simulink model "Complete_Electrolyzer"  (R2022a)
settings: Solver=ode4  StartTime=0.0  StopTime=60  FixedStep=1e-6  RelTol=1e-4
undefined symbols (not defined in the file or in its folder): DiscIntNeverNeededParam
libraries: spsMeanLib x2, spsDCVoltageSourceLib x1, spsControlledCurrentSourceLib x1, spsControlledVoltageSourceLib x1, spsCurrentMeasurementLib x1, spsDiodeLib x1, spsMosfetLib x1, spsVoltageMeasurementLib x1, spspowerguiLib x1
settings Model: Creator=Nikos  LastModifiedBy=nikos
settings SolverCC: MaxConsecutiveZCs=1  ZeroCrossAlgorithm=Adaptive
settings DebuggingCC: IgnoredZcDiagnostic=none

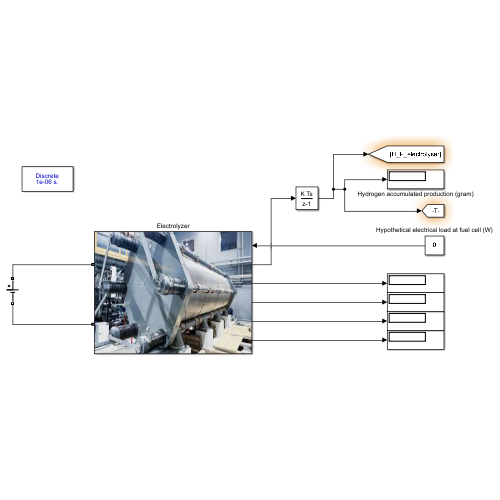
[thumbnail: Simulink's stored preview of the top-level diagram]
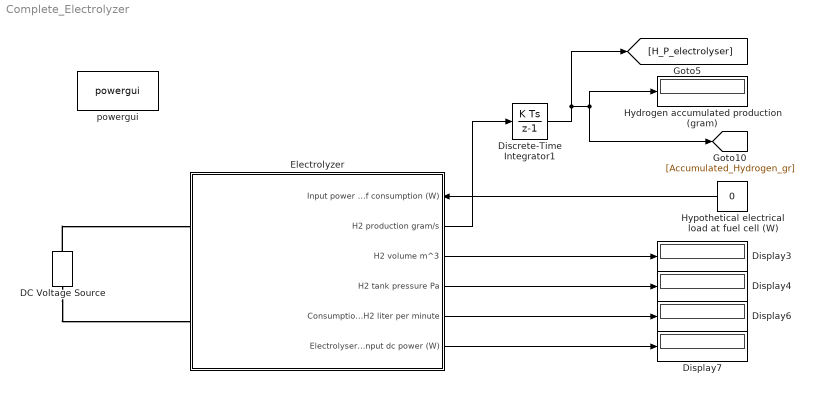
== system Complete_Electrolyzer ==
  DC Voltage Source : spsDCVoltageSourceLib/DC Voltage Source  Amplitude=50  Measurements=None
  Discrete-Time Integrator1 : DiscreteIntegrator  SampleTime=1e-6  ICPrevOutput=DiscIntNeverNeededParam  ICPrevScaledInput=DiscIntNeverNeededParam
  Display{3..4,6..7} (4 alike) : Display
  Electrolyzer : Subsystem
      settings: PortSchema="{\"entries\":[{\"content\":{\"sides\":[{\"content\":{\"connectorIds\":[\"In1\",\"Out1\",\"Out2\",\"Out3\",\"Out4\",\"Out5\"]},\"type\":\"ConnectorPlacement.EquallySpacedRectSide\",\"uuid\":\"586e2a01-0b83-4db1-b05b-c9425d179327\"},{\"content\":{\"connectorIds\":[\"RConn1\",\"RConn2\"],\"side\":\"RIGHT\"},\"type\":\"ConnectorPlacement.EquallySpacedRectSide\",\"uuid\":\"98998693-1c1d-43a0-8265-c06eb7552525\"},{\"content\":{\"connectorIds\":[],\"side\":\"TOP\"},\"type\":\"ConnectorPlacement.EquallySpacedRectSide\",\"uuid\":\"57c96d85-f297-491e-8250-1f4aa33eee63\"}]},\"type\":\"ConnectorPlacement.EquallySpacedConnector\",\"uuid\":\"2efb03bc-2da9-4118-9dbe-8a463fcc009b\"}],\"packageUris\":[\"http://schema.mathworks.com/mf0/Connector/R2020b\"],\"version\":\"1.0\"}"
      mask Display: image('$imagefile'); % Use "Edit Image" on toolstrip to change.
  Hydrogen accumulated production (gram) : Display
  Hypothetical electrical load at fuel cell (W) : Constant  Value=0
  powergui : spspowerguiLib/powergui  Priority=1  SimulationMode=Discrete  SampleTime=1e-6  frequency=60  Iterations=50  frequencyindice=0  Pbase=100e6  ErrMax=1e-4  UnitsV=kV  UnitsW=MW  buscounter=0  FunctionMessages=off  echomessages=off  EnableUseOfTLC=off  CurrentSourceSwitches=off  DisableSnubberDevices=off  DisableRonSwitches=off  DisableVfSwitches=off  DisplayEquations=off  AutomaticDiscreteSolvers=off  SolverType=Tustin/Backward Euler (TBE)  Interpol=off  ExternalGateDelay=off  methode=off  Ts=100  x0status=blocks  SPID=on  SwTol=0  HookPort=off  NonlinearTolerance=1e-4  nMaxIteration=100  ContinueOnMaxIteration=off  RestoreLinks=warning  ResistiveCurrentMeasurement=off  Frange=[0:2:500]  Ylog=off  Xlog=on  ShowGrid=off  save=off  variable=ZData  structure=0  ZoomFFT=off  StartTime=0.0  cycles=1  DisplayStyle=1  fundamental=60  FreqAxis=off  MaxFrequency=1000  frequencyindicesteady=1  RmsSteady=1  display=off
  wires:
  Electrolyzer/2(H2 volume m^3) -> Display3/1
  Electrolyzer/4(Consumption of H2 liter per minute) -> Display6/1
  Electrolyzer/5(Electrolyser input dc power (W)) -> Display7/1
  Electrolyzer/3(H2 tank pressure Pa) -> Display4/1
  Discrete-Time Integrator1/1 -> [H_P_electrolyser], [Accumulated_Hydrogen_gr], Hydrogen accumulated production (gram)/1
  Electrolyzer/1(H2 production gram/s) -> Discrete-Time Integrator1/1
  Hypothetical electrical load at fuel cell (W)/1 -> Electrolyzer/1(Input power of consumption (W))
  connections:
  DC Voltage Source/RConn1 -- Electrolyzer/RConn1
  DC Voltage Source/LConn1 -- Electrolyzer/RConn2

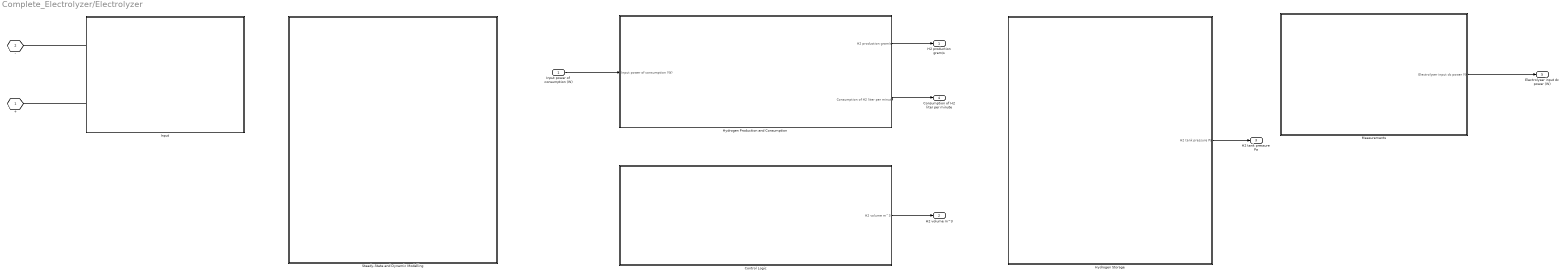
== system Complete_Electrolyzer/Electrolyzer ==
  Input power of consumption (W) : Inport
  Control Logic : Subsystem
  Hydrogen Production and Consumption : Subsystem
  Hydrogen Storage : Subsystem
  Input : Subsystem
  Measurements : Subsystem
  Steady-State and Dynamic Modelling : Subsystem
  + : PMIOPort  Tag=PMCPort  Side=Right
  - : PMIOPort  Tag=PMCPort  Port=2  Side=Right
  H2 production gram/s : Outport
  H2 volume m^3 : Outport  Port=2
  H2 tank pressure Pa : Outport  Port=3
  Consumption of H2 liter per minute : Outport  Port=4
  Electrolyser input dc power (W) : Outport  Port=5
  wires:
  Input power of consumption (W)/1 -> Hydrogen Production and Consumption/1(Input power of consumption (W))
  Hydrogen Production and Consumption/1(H2 production gram/s) -> H2 production gram/s/1
  Hydrogen Production and Consumption/2(Consumption of H2 liter per minute) -> Consumption of H2 liter per minute/1
  Control Logic/1(H2 volume m^3) -> H2 volume m^3/1
  Hydrogen Storage/1(H2 tank pressure Pa) -> H2 tank pressure Pa/1
  Measurements/1(Electrolyser input dc power (W)) -> Electrolyser input dc power (W)/1
  connections:
  Input/RConn1 -- -/RConn1
  Input/RConn2 -- +/RConn1

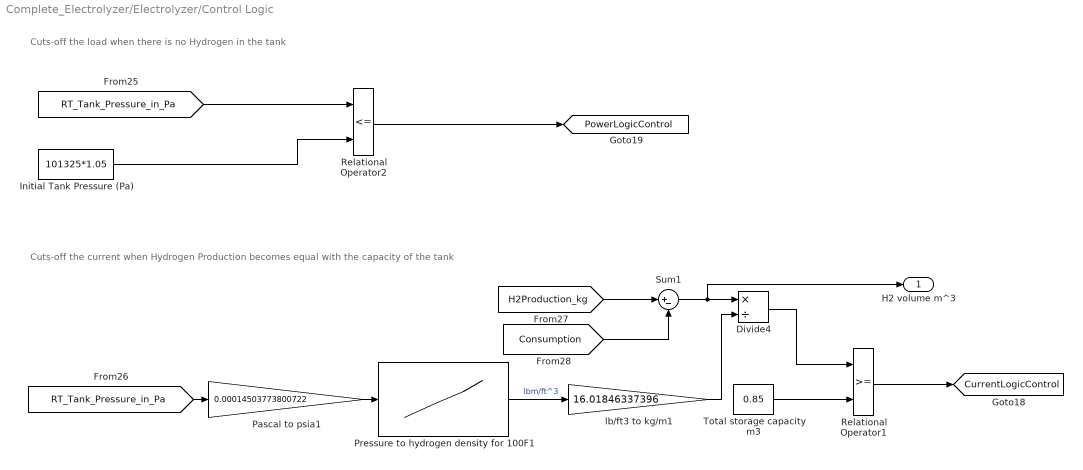
== system Complete_Electrolyzer/Electrolyzer/Control Logic ==
  note: Cuts-off the load when there is no Hydrogen in the tank
  note: Cuts-off the current when Hydrogen Production becomes equal with the capacity of the tank
  Divide4 : Product  Inputs=*/
  Initial Tank Pressure (Pa) : Constant  Value=101325*1.05
  Pascal to psia1 : Gain  Gain=0.00014503773800722
  Pressure to hydrogen density for 100F1 : Lookup_n-D  NumberOfTableDimensions=1  BreakpointsForDimension1=[5 50 100 500 1000 2000 5000 10000]  Table=[0.0017 0.0167 0.0334 0.1646 0.3228 0.6209 1.3875 2.3522]  InternalRulePriority=Speed  RndMeth=Simplest
  Relational Operator1 : RelationalOperator  OutDataTypeStr=boolean  RndMeth=Simplest  InputSameDT=off
  Relational Operator2 : RelationalOperator  Operator=<=  OutDataTypeStr=boolean  RndMeth=Simplest  InputSameDT=off
  Sum1 : Sum  Inputs=|+-
  Total storage capacity m3 : Constant  Value=0.85
  lb/ft3 to kg/m1 : Gain  Gain=16.01846337396
  H2 volume m^3 : Outport
  tag scope: CurrentLogicControl=global, PowerLogicControl=global
  wires:
  [H2Production_kg] -> Sum1/1
  Relational Operator1/1 -> [CurrentLogicControl]
  Sum1/1 -> H2 volume m^3/1, Divide4/1
  Initial Tank Pressure (Pa)/1 -> Relational Operator2/2
  Relational Operator2/1 -> [PowerLogicControl]
  Pascal to psia1/1 -> Pressure to hydrogen density for 100F1/1
  Pressure to hydrogen density for 100F1/1 -> lb/ft3 to kg/m1/1  "lbm/ft^3"
  lb/ft3 to kg/m1/1 -> Divide4/2
  Divide4/1 -> Relational Operator1/1
  Total storage capacity m3/1 -> Relational Operator1/2
  [RT_Tank_Pressure_in_Pa] -> Pascal to psia1/1
  [Consumption] -> Sum1/2
  [RT_Tank_Pressure_in_Pa] -> Relational Operator2/1

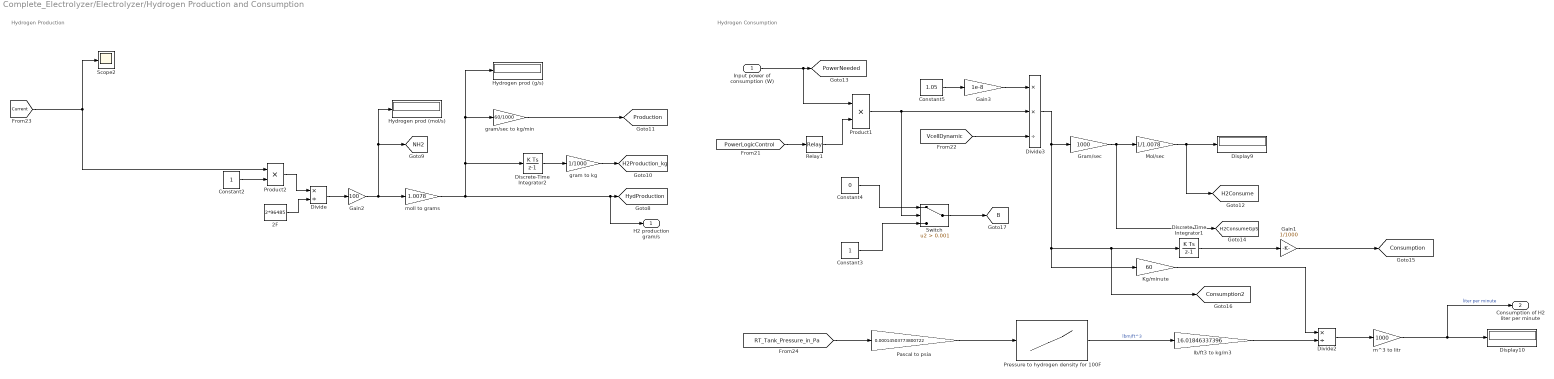
== system Complete_Electrolyzer/Electrolyzer/Hydrogen Production and Consumption ==
  note: Hydrogen Production
  note: Hydrogen Consumption
  Input power of consumption (W) : Inport
  2F : Constant  Value=2*96485
  Constant2 : Constant
  Constant3 : Constant
  Constant4 : Constant  Value=0
  Constant5 : Constant  Value=1.05
  Discrete-Time Integrator1 : DiscreteIntegrator  SampleTime=1e-6  ICPrevOutput=DiscIntNeverNeededParam  ICPrevScaledInput=DiscIntNeverNeededParam
  Discrete-Time Integrator2 : DiscreteIntegrator  SampleTime=1e-6  ICPrevOutput=DiscIntNeverNeededParam  ICPrevScaledInput=DiscIntNeverNeededParam
  Display10 : Display
  Display9 : Display
  Divide : Product  Inputs=*/
  Divide2 : Product  Inputs=*/
  Divide3 : Product  Inputs=**/
  Gain1 : Gain  Gain=1/1000
  Gain2 : Gain  Gain=100
  Gain3 : Gain  Gain=1e-8
  Gram/sec : Gain  Gain=1000
  Hydrogen prod (g/s) : Display
  Hydrogen prod (mol/s) : Display
  Kg/minute : Gain  Gain=60
  Mol/sec : Gain  Gain=1/1.0078
  Pascal to psia : Gain  Gain=0.00014503773800722
  Pressure to hydrogen density for 100F : Lookup_n-D  NumberOfTableDimensions=1  BreakpointsForDimension1=[5 50 100 500 1000 2000 5000 10000]  Table=[0.0017 0.0167 0.0334 0.1646 0.3228 0.6209 1.3875 2.3522]  InternalRulePriority=Speed  RndMeth=Simplest
  Product1 : Product
  Product2 : Product
  Relay1 : Relay  OnOutputValue=0  OffOutputValue=1
  Scope2 : Scope
  Switch : Switch  Criteria=u2 > Threshold  Threshold=0.001  SaturateOnIntegerOverflow=off  InputSameDT=off
  gram to kg : Gain  Gain=1/1000
  gram/sec to kg/min : Gain  Gain=60/1000
  lb/ft3 to kg/m3 : Gain  Gain=16.01846337396
  m^3 to litr : Gain  Gain=1000
  moll to grams : Gain  Gain=1.0078
  H2 production gram/s : Outport
  Consumption of H2 liter per minute : Outport  Port=2
  tag scope: B=global, Consumption2=global, Consumption=global, H2Consume=global, H2ConsumeGpS=global, H2Production_kg=global, HydProduction=global, NH2=global, PowerNeeded=global, Production=global
  wires:
  Input power of consumption (W)/1 -> Product1/1, [PowerNeeded]
  Relay1/1 -> Product1/2
  Divide3/1 -> [Consumption2], Discrete-Time Integrator1/1, Kg/minute/1, Gram/sec/1
  [VcellDynamic] -> Divide3/3
  Divide/1 -> Gain2/1
  Gram/sec/1 -> [H2ConsumeGpS], Mol/sec/1
  Mol/sec/1 -> [H2Consume], Display9/1
  Gain2/1 -> [NH2], Hydrogen prod (mol/s)/1, moll to grams/1
  Pascal to psia/1 -> Pressure to hydrogen density for 100F/1
  Discrete-Time Integrator1/1 -> Gain1/1
  moll to grams/1 -> Hydrogen prod (g/s)/1, gram/sec to kg/min/1, Discrete-Time Integrator2/1, H2 production gram/s/1, [HydProduction]
  Product1/1 -> Switch/2, Divide3/2
  m^3 to litr/1 -> Consumption of H2 liter per minute/1, Display10/1  "liter per minute"
  Pressure to hydrogen density for 100F/1 -> lb/ft3 to kg/m3/1  "lbm/ft^3"
  [PowerLogicControl] -> Relay1/1
  [Current] -> Scope2/1, Product2/1
  Constant5/1 -> Gain3/1
  Kg/minute/1 -> Divide2/1
  [RT_Tank_Pressure_in_Pa] -> Pascal to psia/1
  Gain1/1 -> [Consumption]
  Gain3/1 -> Divide3/1
  Constant3/1 -> Switch/3
  lb/ft3 to kg/m3/1 -> Divide2/2
  Constant4/1 -> Switch/1
  gram to kg/1 -> [H2Production_kg]
  gram/sec to kg/min/1 -> [Production]
  Divide2/1 -> m^3 to litr/1
  Product2/1 -> Divide/1
  2F/1 -> Divide/2
  Switch/1 -> [B]
  Constant2/1 -> Product2/2
  Discrete-Time Integrator2/1 -> gram to kg/1

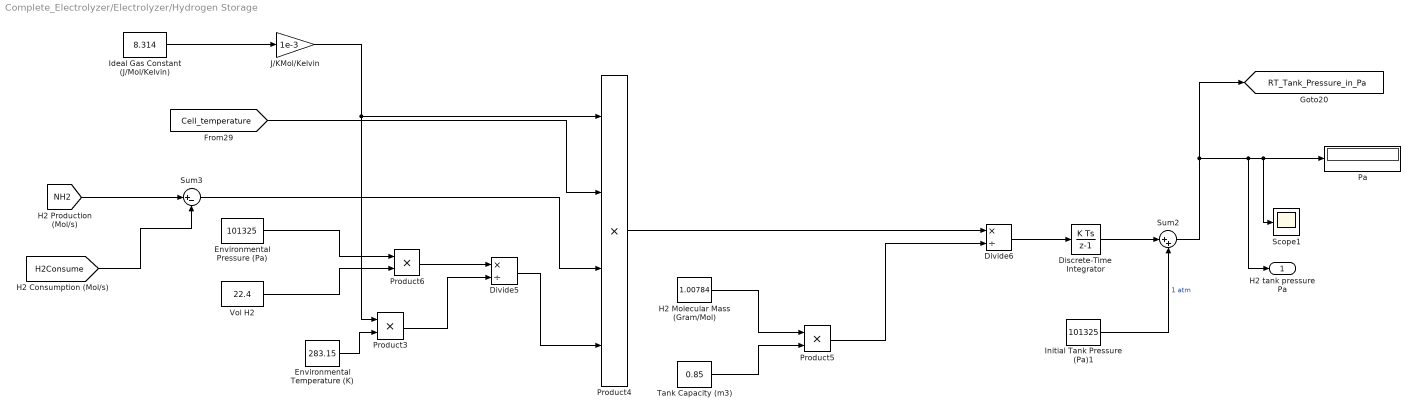
== system Complete_Electrolyzer/Electrolyzer/Hydrogen Storage ==
  Discrete-Time Integrator : DiscreteIntegrator  SampleTime=1e-6  ICPrevOutput=DiscIntNeverNeededParam  ICPrevScaledInput=DiscIntNeverNeededParam
  Divide5 : Product  Inputs=*/
  Divide6 : Product  Inputs=*/
  Environmental Pressure (Pa) : Constant  Value=101325
  Environmental Temperature (K) : Constant  Value=283.15
  H2 Molecular Mass (Gram/Mol) : Constant  Value=1.00784
  Ideal Gas Constant (J/Mol/Kelvin) : Constant  Value=8.314
  Initial Tank Pressure (Pa)1 : Constant  Value=101325
  J/KMol/Kelvin : Gain  Gain=1e-3
  Pa : Display
  Product3 : Product
  Product4 : Product  Inputs=4
  Product5 : Product
  Product6 : Product
  Scope1 : Scope
  Sum2 : Sum  Inputs=|++
  Sum3 : Sum  Inputs=|+-
  Tank Capacity (m3) : Constant  Value=0.85
  Vol H2 : Constant  Value=22.4
  H2 tank pressure Pa : Outport
  tag scope: RT_Tank_Pressure_in_Pa=global
  wires:
  Environmental Temperature (K)/1 -> Product3/2
  J/KMol/Kelvin/1 -> Product4/1, Product3/1
  Product3/1 -> Divide5/2
  Discrete-Time Integrator/1 -> Sum2/1
  [H2Consume] -> Sum3/2
  Sum3/1 -> Product4/3
  Product6/1 -> Divide5/1
  Divide6/1 -> Discrete-Time Integrator/1
  Vol H2/1 -> Product6/2
  Tank Capacity (m3)/1 -> Product5/2
  Sum2/1 -> [RT_Tank_Pressure_in_Pa], H2 tank pressure Pa/1, Scope1/1, Pa/1
  Environmental Pressure (Pa)/1 -> Product6/1
  Ideal Gas Constant (J/Mol/Kelvin)/1 -> J/KMol/Kelvin/1
  Product5/1 -> Divide6/2
  Divide5/1 -> Product4/4
  H2 Molecular Mass (Gram/Mol)/1 -> Product5/1
  Product4/1 -> Divide6/1
  [NH2] -> Sum3/1
  [Cell_temperature] -> Product4/2
  Initial Tank Pressure (Pa)1/1 -> Sum2/2  "1 atm"

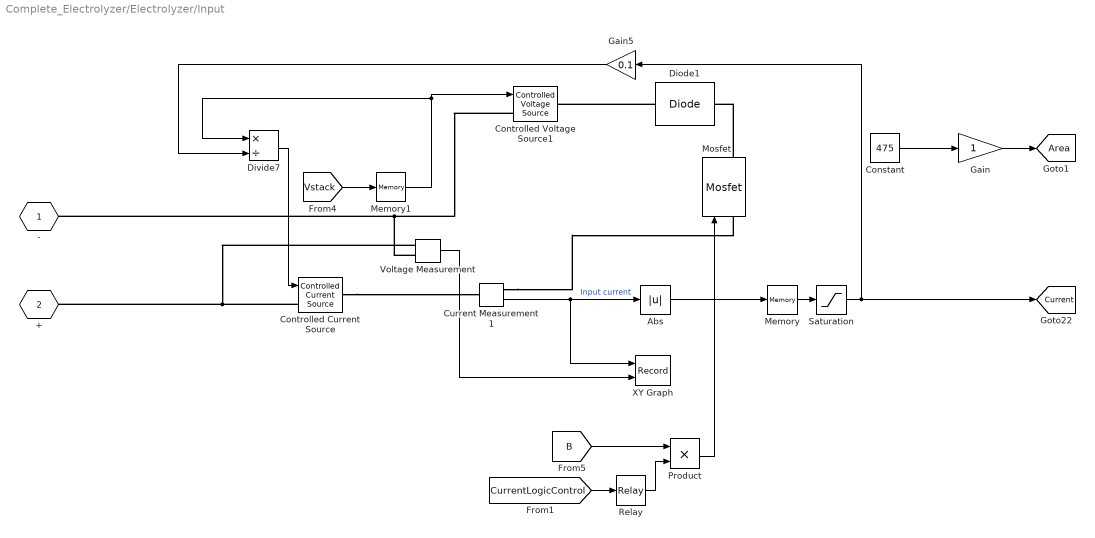
== system Complete_Electrolyzer/Electrolyzer/Input ==
  Abs : Abs  SaturateOnIntegerOverflow=off
  Constant : Constant  Value=475
  Controlled Current Source : spsControlledCurrentSourceLib/Controlled Current Source  Initialize=off  Source_Type=DC  Amplitude=0  Phase=0  Frequency=0  Measurements=None
  Controlled Voltage Source1 : spsControlledVoltageSourceLib/Controlled Voltage Source  Initialize=off  Source_Type=DC  Amplitude=0  Phase=0  Frequency=0  Measurements=None
  Current Measurement1 : spsCurrentMeasurementLib/Current Measurement  PhasorSimulation=off  OutputType=Complex  PSBequivalent=0
  Diode1 : spsDiodeLib/Diode  Ron=0.001  Lon=0  Vf=0  IC=0  UseSnubber=0  Rs=10e6  Cs=inf  Measurements=off
  Divide7 : Product  Inputs=*/
  Gain : Gain
  Gain5 : Gain  Gain=0.1
  Memory : Memory  InitialCondition=6  InheritSampleTime=on
  Memory1 : Memory  InitialCondition=6  InheritSampleTime=on
  Mosfet : spsMosfetLib/Mosfet  Ron=0.000001  Lon=0  Rd=0.01  Vfd=0  IC=0  Rs=1e-6  Cs=inf  Measurements=on
  Product : Product
  Relay : Relay  OnOutputValue=0  OffOutputValue=1
  Saturation : Saturate  UpperLimit=25  LowerLimit=0
  Voltage Measurement : spsVoltageMeasurementLib/Voltage Measurement  PhasorSimulation=off  OutputType=Complex  PSBequivalent=0
  XY Graph : Record  FileSettingsInternal="{\"entries\":[{\"content\":{\"excelSettings\":{\"content\":{},\"type\":\"Streamout.ExcelSettings\"}},\"type\":\"Streamout.FileSettingStorage\",\"uuid\":\"27254736-f3cb-41f8-afc9-4dd85544c286\"}],\"packageUris\":[\"http://schema.mathworks.com/mf0/streamout_blocks/R2020a\"],\"version\":\"1.0\"}"  Layout=[1 1]  SignalsInternal="{\"entries\":[{\"content\":{\"signals\":[{\"content\":{\"blockPath\":[\"Complete_Electrolyzer/Electrolyzer/Input/XY Graph\"],\"channel\":[],\"dimensions\":[1],\"domain\":\"Complete_Electrolyzer/Electrolyzer/Input/XY Graph\",\"lineColor\":\"#a2142f\",\"plots\":[1],\"port\":1,\"sid\":[],\"signalID\":9,\"signalName\":\"Input current\"},\"type\":\"RecordBlkView.Signal\",\"uuid\":\"a5d2c1d2-6a3b-4fd5-9de4-d17e008494c7\"},{\"content\":{\"blockPath\":[\"Complete_Electrolyzer/Electrolyzer/Input/XY Graph\"],\"channel\":[],\"dimensions\":[1],\"domain\":\"Complete_Electrolyzer/Electrolyzer/Input/XY Graph\",\"lineColor\":\"#139fff\",\"plots\":[1],\"port\":2,\"sid\":[],\"signalID\":12,\"signalName\":\"Voltage Measurement\"},\"type\":\"RecordBlkView.Signal\",\"uuid\":\"0852a48e-418c-4982-9cdf-9d86dec133ab\"}]},\"type\":\"RecordBlkView.InputSignals\",\"uuid\":\"9df3a92c-e0b3-4336-b1e3-4f5ec8f4d684\"}],\"packageUris\":[\"http://schema.mathworks.com/mf0/streamout_blocks/R2020a\"],\"version\":\"1.0\"}"  VisualizationBindings="{\"xyplotplugin\":{\"info\":[{\"series\":[{\"bindingParametersList\":[{\"parameter\":\"X-Axis\",\"signalID\":9,\"signalName\":\"Input current\"},{\"parameter\":\"Y-Axis\",\"signalID\":12,\"signalName\":\"Voltage Measurement\"}],\"seriesID\":43300}],\"subplotID\":1}]}}"  CompatibilityTag=XY
  - : PMIOPort  Tag=PMCPort  Side=Right
  + : PMIOPort  Tag=PMCPort  Port=2  Side=Right
  tag scope: Area=global, Current=global
  wires:
  Gain5/1 -> Divide7/2
  [CurrentLogicControl] -> Relay/1
  Memory/1 -> Saturation/1
  Constant/1 -> Gain/1
  Memory1/1 -> Divide7/1, Controlled Voltage Source1/1
  Relay/1 -> Product/2
  Voltage Measurement/1 -> XY Graph/2
  Saturation/1 -> [Current], Gain5/1
  Gain/1 -> [Area]
  [B] -> Product/1
  Current Measurement1/1 -> Abs/1, XY Graph/1  "Input current"
  [Vstack] -> Memory1/1
  Abs/1 -> Memory/1
  Product/1 -> Mosfet/1
  Divide7/1 -> Controlled Current Source/1
  connections:
  Voltage Measurement/LConn1 -- Controlled Current Source/LConn1 -- +/RConn1
  Diode1/RConn1 -- Controlled Voltage Source1/RConn1
  Voltage Measurement/LConn2 -- Controlled Voltage Source1/LConn1 -- -/RConn1
  Controlled Current Source/RConn1 -- Current Measurement1/LConn1
  Mosfet/RConn1 -- Diode1/LConn1
  Current Measurement1/RConn1 -- Mosfet/LConn1

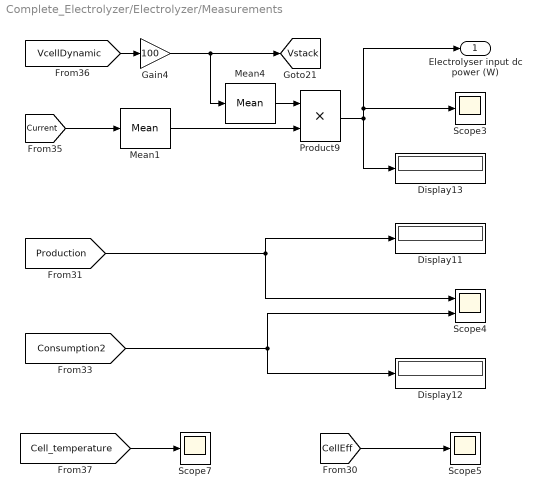
== system Complete_Electrolyzer/Electrolyzer/Measurements ==
  Display11 : Display
  Display12 : Display
  Display13 : Display
  Gain4 : Gain  Gain=100
  Mean1 : spsMeanLib/Mean  Freq=50  Vinit=0  Ts=1e-6
  Mean4 : spsMeanLib/Mean  Freq=50  Vinit=0  Ts=1e-6
  Product9 : Product
  Scope3 : Scope
  Scope4 : Scope  NumInputPorts=2
  Scope5 : Scope
  Scope7 : Scope
  Electrolyser input dc power (W) : Outport
  tag scope: Vstack=global
  wires:
  [Consumption2] -> Scope4/2, Display12/1
  [Cell_temperature] -> Scope7/1
  [VcellDynamic] -> Gain4/1
  Mean1/1 -> Product9/2
  Mean4/1 -> Product9/1
  Product9/1 -> Electrolyser input dc power (W)/1, Scope3/1, Display13/1
  [CellEff] -> Scope5/1
  Gain4/1 -> [Vstack], Mean4/1
  [Production] -> Display11/1, Scope4/1
  [Current] -> Mean1/1

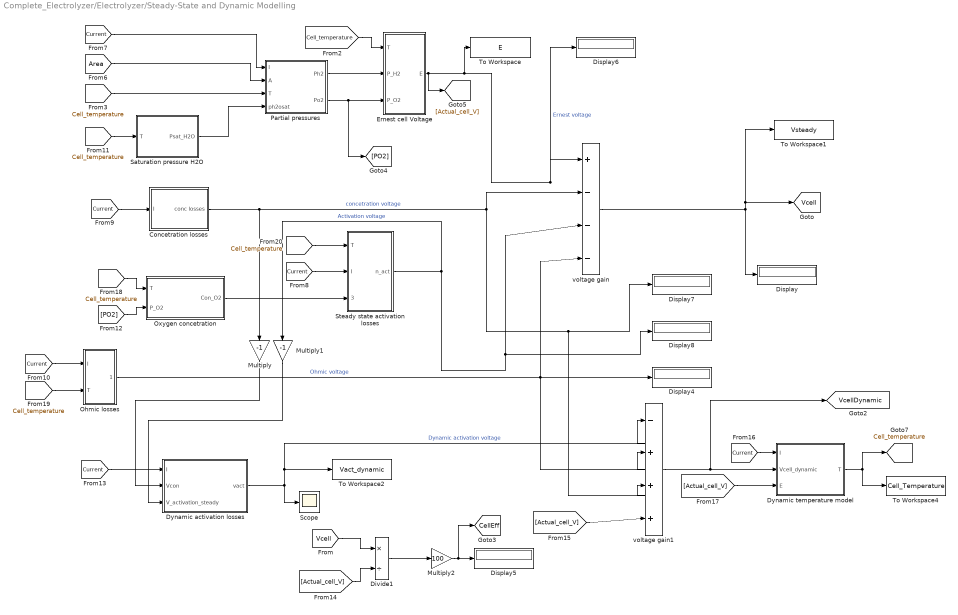
== system Complete_Electrolyzer/Electrolyzer/Steady-State and Dynamic Modelling ==
  " voltage gain" : Sum  Inputs=|+---
  " voltage gain1" : Sum  Inputs=|-+++
  Concetration losses : Subsystem
  Display{,4..8} (6 alike) : Display
  Divide1 : Product  Inputs=*/
  Dynamic activation losses : Subsystem
  Dynamic temperature model : Subsystem
  Ernest cell Voltage : Subsystem
  Multiply : Gain  Gain=-1
  Multiply1 : Gain  Gain=-1
  Multiply2 : Gain  Gain=100
  Ohmic losses : Subsystem
  Oxygen concetration : Subsystem
  Partial pressures : Subsystem
  Saturation pressure H2O : Subsystem
  Scope : Scope
  Steady state activation losses : Subsystem
  To Workspace : ToWorkspace  VariableName=E  SampleTime=-1
  To Workspace1 : ToWorkspace  VariableName=Vsteady  SaveFormat=Timeseries  SampleTime=-1
  To Workspace2 : ToWorkspace  VariableName=Vact_dynamic  SaveFormat=Timeseries  SampleTime=-1
  To Workspace4 : ToWorkspace  VariableName=Cell_Temperature  SaveFormat=Structure With Time  SampleTime=-1
  tag scope: CellEff=global, Cell_temperature=global, Vcell=global, VcellDynamic=global
  wires:
  " voltage gain1"/1 -> Dynamic temperature model/2(Vcell_dynamic), [VcellDynamic]
  Concetration losses/1(conc losses) -> " voltage gain1"/3, Display7/1, " voltage gain"/2, Multiply/1  "concetration voltage"
  [Vcell] -> Divide1/1
  Ohmic losses/1(nohm) -> " voltage gain1"/2, Display4/1, " voltage gain"/4  "Ohmic voltage"
  Dynamic activation losses/1(vact) -> Scope/1, " voltage gain1"/1, To Workspace2/1  "Dynamic activation voltage"
  " voltage gain"/1 -> [Vcell], To Workspace1/1, Display/1
  Divide1/1 -> Multiply2/1
  [Cell_temperature] -> Saturation pressure H2O/1(T)
  Steady state activation losses/1(n_act) -> Display8/1, " voltage gain"/3, Multiply1/1  "Activation voltage"
  [Current] -> Dynamic temperature model/1(I)
  [Current] -> Partial pressures/1(I)
  Ernest cell Voltage/1(E) -> To Workspace/1, Display6/1, " voltage gain"/1, [Actual_cell_V]  "Ernest voltage"
  [Current] -> Ohmic losses/1(I)
  [Cell_temperature] -> Ohmic losses/2(T)
  [Cell_temperature] -> Partial pressures/3(T)
  [Actual_cell_V] -> Dynamic temperature model/3(E)
  [Cell_temperature] -> Steady state activation losses/1(T)
  Saturation pressure H2O/1(Psat_H2O) -> Partial pressures/4(ph2osat)
  Partial pressures/2(Po2) -> Ernest cell Voltage/3(P_O2), [PO2]
  Multiply1/1 -> Dynamic activation losses/3(V_activation_steady)
  [Current] -> Steady state activation losses/2(I)
  Partial pressures/1(Ph2) -> Ernest cell Voltage/2(P_H2)
  [Cell_temperature] -> Oxygen concetration/1(T)
  Dynamic temperature model/1(T) -> To Workspace4/1, [Cell_temperature]
  [PO2] -> Oxygen concetration/2(P_O2)
  [Actual_cell_V] -> " voltage gain1"/4
  [Current] -> Concetration losses/1(I)
  Multiply/1 -> Dynamic activation losses/2(Vcon)
  [Current] -> Dynamic activation losses/1(I)
  [Cell_temperature] -> Ernest cell Voltage/1(T)
  Oxygen concetration/1(Con_O2) -> Steady state activation losses/3(Con_O2)
  [Area] -> Partial pressures/2(A)
  [Actual_cell_V] -> Divide1/2
  Multiply2/1 -> [CellEff], Display5/1

== system Complete_Electrolyzer/Electrolyzer/Steady-State and Dynamic Modelling/Concetration losses ==
  I : Inport
  . : Sum  Inputs=|-+
  B : Constant  Value=0.016
  Constant3 : Constant
  Divide2 : Product  Inputs=*/
  Exp : Math  Operator=log
  Product : Product
  limiting current : Constant  Value=25.1
  conc losses : Outport
  wires:
  Exp/1 -> Product/1
  Product/1 -> conc losses/1
  Constant3/1 -> ./2
  B/1 -> Product/2
  Divide2/1 -> ./1
  limiting current/1 -> Divide2/2
  I/1 -> Divide2/1
  ./1 -> Exp/1

== system Complete_Electrolyzer/Electrolyzer/Steady-State and Dynamic Modelling/Dynamic activation losses ==
  I : Inport
  Vcon : Inport  Port=2
  V_activation_steady : Inport  Port=3
  . : Sum  Inputs=|++
  .1 : Sum  Inputs=|+-
  Constant : Constant
  Discrete-Time Integrator : DiscreteIntegrator  SampleTime=1e-6  ICPrevOutput=DiscIntNeverNeededParam  ICPrevScaledInput=DiscIntNeverNeededParam
  Divide1 : Product  Inputs=*/
  Divide2 : Product  Inputs=/*
  Divide3 : Product  Inputs=/*
  Product : Product
  vact : Outport
  wires:
  ./1 -> Divide2/2
  Discrete-Time Integrator/1 -> Divide3/2, vact/1
  I/1 -> Divide1/1, Divide2/1
  Divide1/1 -> .1/1
  .1/1 -> Discrete-Time Integrator/1
  Constant/1 -> Product/1, Divide1/2
  V_activation_steady/1 -> ./2
  Vcon/1 -> ./1
  Divide2/1 -> Product/2
  Divide3/1 -> .1/2
  Product/1 -> Divide3/1

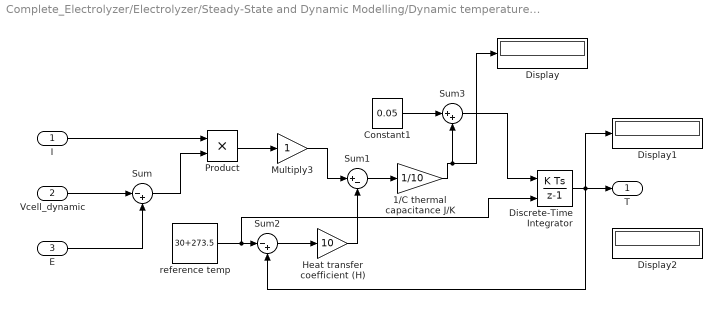
== system Complete_Electrolyzer/Electrolyzer/Steady-State and Dynamic Modelling/Dynamic temperature model ==
  I : Inport
  Vcell_dynamic : Inport  Port=2
  E : Inport  Port=3
  1/C thermal capacitance J/K : Gain  Gain=1/10
  Constant1 : Constant  Value=0.05
  Discrete-Time Integrator : DiscreteIntegrator  InitialConditionSource=external  InitialCondition=0.001  SampleTime=1e-6  ICPrevOutput=DiscIntNeverNeededParam  ICPrevScaledInput=DiscIntNeverNeededParam
  Display : Display
  Display1 : Display
  Display2 : Display
  Heat transfer coefficient (H) : Gain  Gain=10
  Multiply3 : Gain
  Product : Product
  Sum : Sum  Inputs=|-+
  Sum1 : Sum  Inputs=|+-
  Sum2 : Sum  Inputs=|-+
  Sum3 : Sum  Inputs=|++
  reference temp : Constant  Value=30+273.5
  T : Outport
  wires:
  Multiply3/1 -> Sum1/1
  Product/1 -> Multiply3/1
  Discrete-Time Integrator/1 -> Sum2/2, Display1/1, T/1
  Sum2/1 -> Heat transfer coefficient (H)/1
  I/1 -> Product/1
  Vcell_dynamic/1 -> Sum/1
  Sum/1 -> Product/2
  E/1 -> Sum/2
  Sum1/1 -> 1/C thermal capacitance J/K/1
  Heat transfer coefficient (H)/1 -> Sum1/2
  reference temp/1 -> Discrete-Time Integrator/2, Sum2/1
  1/C thermal capacitance J/K/1 -> Display/1, Sum3/2
  Constant1/1 -> Sum3/1
  Sum3/1 -> Discrete-Time Integrator/1

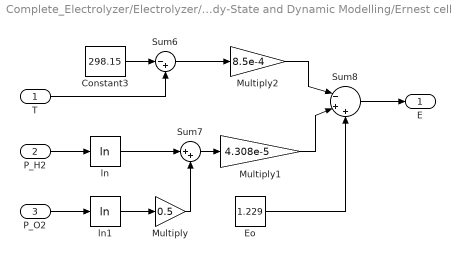
== system Complete_Electrolyzer/Electrolyzer/Steady-State and Dynamic Modelling/Ernest cell Voltage ==
  T : Inport
  P_H2 : Inport  Port=2
  P_O2 : Inport  Port=3
  Constant3 : Constant  Value=298.15
  Eo : Constant  Value=1.229
  Multiply : Gain  Gain=0.5
  Multiply1 : Gain  Gain=4.308e-5
  Multiply2 : Gain  Gain=8.5e-4
  Sum6 : Sum  Inputs=|-+
  Sum7 : Sum  Inputs=|++
  Sum8 : Sum  Inputs=|-++
  ln : Math  Operator=log
  ln1 : Math  Operator=log
  E : Outport
  wires:
  Constant3/1 -> Sum6/1
  Sum6/1 -> Multiply2/1
  ln1/1 -> Multiply/1
  Eo/1 -> Sum8/3
  Multiply1/1 -> Sum8/2
  Sum8/1 -> E/1
  Sum7/1 -> Multiply1/1
  Multiply/1 -> Sum7/2
  P_H2/1 -> ln/1
  T/1 -> Sum6/2
  ln/1 -> Sum7/1
  P_O2/1 -> ln1/1
  Multiply2/1 -> Sum8/1

== system Complete_Electrolyzer/Electrolyzer/Steady-State and Dynamic Modelling/Ohmic losses ==
  I : Inport
  T : Inport  Port=2
  . : Sum  Inputs=|+-+
  Constant3 : Constant  Value=1.605e-2
  Multiply : Gain  Gain=8e-5
  Multiply1 : Gain  Gain=3.5e-5
  Multiply2 : Gain  Gain=-1
  Product : Product
  nohm : Outport
  wires:
  Product/1 -> nohm/1
  Multiply1/1 -> ./2
  I/1 -> Multiply2/1, Multiply/1
  Multiply/1 -> ./1
  Multiply2/1 -> Product/1
  ./1 -> Product/2
  Constant3/1 -> ./3
  T/1 -> Multiply1/1

== system Complete_Electrolyzer/Electrolyzer/Steady-State and Dynamic Modelling/Oxygen concetration ==
  T : Inport
  P_O2 : Inport  Port=2
  Constant3 : Constant  Value=-498
  Constant4 : Constant  Value=5.08e6
  Divide1 : Product  Inputs=/*
  Divide2 : Product  Inputs=*/
  Exp : Math
  Product : Product
  Con_O2 : Outport
  wires:
  Exp/1 -> Product/1
  P_O2/1 -> Divide1/2
  Constant3/1 -> Divide2/1
  Divide1/1 -> Con_O2/1
  T/1 -> Divide2/2
  Constant4/1 -> Product/2
  Product/1 -> Divide1/1
  Divide2/1 -> Exp/1

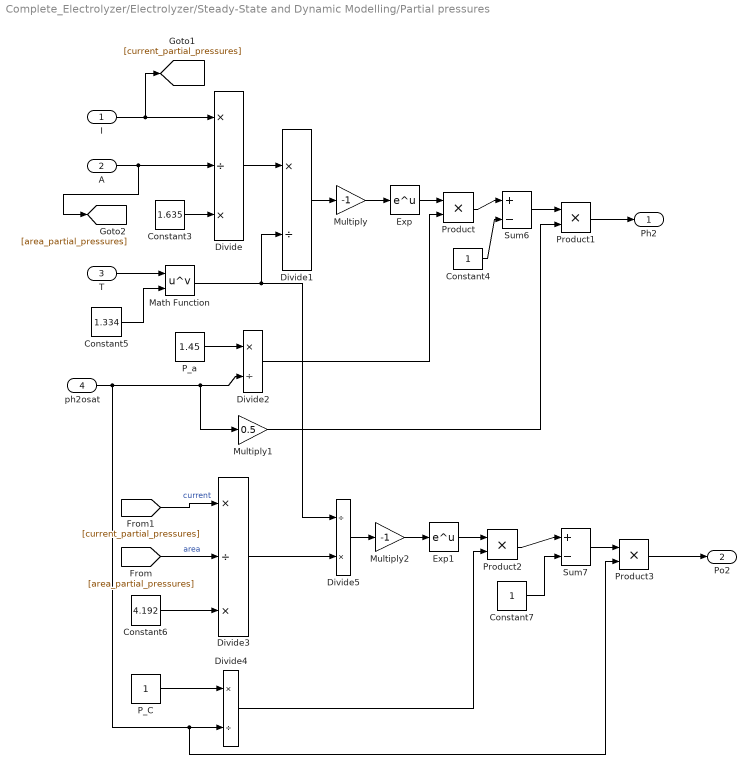
== system Complete_Electrolyzer/Electrolyzer/Steady-State and Dynamic Modelling/Partial pressures ==
  I : Inport
  A : Inport  Port=2
  T : Inport  Port=3
  ph2osat : Inport  Port=4
  Constant3 : Constant  Value=1.635
  Constant4 : Constant
  Constant5 : Constant  Value=1.334
  Constant6 : Constant  Value=4.192
  Constant7 : Constant
  Divide : Product  Inputs=*/*
  Divide1 : Product  Inputs=*/
  Divide2 : Product  Inputs=*/
  Divide3 : Product  Inputs=*/*
  Divide4 : Product  Inputs=*/
  Divide5 : Product  Inputs=/*
  Exp : Math
  Exp1 : Math
  Math Function : Math  Operator=pow
  Multiply : Gain  Gain=-1
  Multiply1 : Gain  Gain=0.5
  Multiply2 : Gain  Gain=-1
  P_C : Constant
  P_a : Constant  Value=1.45
  Product{,1..3} (4 alike) : Product
  Sum6 : Sum  Inputs=|+-
  Sum7 : Sum  Inputs=|+-
  Ph2 : Outport
  Po2 : Outport  Port=2
  wires:
  Constant5/1 -> Math Function/2
  Constant7/1 -> Sum7/2
  Constant6/1 -> Divide3/3
  Constant4/1 -> Sum6/2
  ph2osat/1 -> Multiply1/1, Divide2/2, Product3/2, Divide4/2
  Divide5/1 -> Multiply2/1
  A/1 -> [area_partial_pressures], Divide/2
  T/1 -> Math Function/1
  Product2/1 -> Sum7/1
  Divide3/1 -> Divide5/2
  Product1/1 -> Ph2/1
  Exp/1 -> Product/1
  Constant3/1 -> Divide/3
  I/1 -> [current_partial_pressures], Divide/1
  Multiply/1 -> Exp/1
  P_C/1 -> Divide4/1
  Math Function/1 -> Divide5/1, Divide1/2
  Sum7/1 -> Product3/1
  [current_partial_pressures] -> Divide3/1  "current"
  Multiply1/1 -> Product1/2
  Multiply2/1 -> Exp1/1
  Exp1/1 -> Product2/1
  Divide1/1 -> Multiply/1
  Divide/1 -> Divide1/1
  Sum6/1 -> Product1/1
  Product/1 -> Sum6/1
  Divide4/1 -> Product2/2
  P_a/1 -> Divide2/1
  [area_partial_pressures] -> Divide3/2  "area"
  Product3/1 -> Po2/1
  Divide2/1 -> Product/2

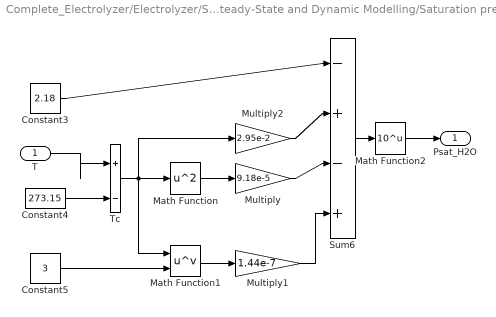
== system Complete_Electrolyzer/Electrolyzer/Steady-State and Dynamic Modelling/Saturation pressure H2O ==
  T : Inport
  Constant3 : Constant  Value=2.18
  Constant4 : Constant  Value=273.15
  Constant5 : Constant  Value=3
  Math Function : Math  Operator=square
  Math Function1 : Math  Operator=pow
  Math Function2 : Math  Operator=10^u
  Multiply : Gain  Gain=9.18e-5
  Multiply1 : Gain  Gain=1.44e-7
  Multiply2 : Gain  Gain=2.95e-2
  Sum6 : Sum  Inputs=|-+-+
  Tc : Sum  Inputs=|+-
  Psat_H2O : Outport
  wires:
  Multiply1/1 -> Sum6/4
  Constant3/1 -> Sum6/1
  Math Function2/1 -> Psat_H2O/1
  Math Function/1 -> Multiply/1
  Constant5/1 -> Math Function1/2
  Tc/1 -> Multiply2/1, Math Function/1, Math Function1/1
  Sum6/1 -> Math Function2/1
  Multiply/1 -> Sum6/3
  T/1 -> Tc/1
  Math Function1/1 -> Multiply1/1
  Multiply2/1 -> Sum6/2
  Constant4/1 -> Tc/2

== system Complete_Electrolyzer/Electrolyzer/Steady-State and Dynamic Modelling/Steady state activation losses ==
  T : Inport
  I : Inport  Port=2
  Con_O2 : Inport  Port=3
  Constant3 : Constant  Value=0.9514
  Exp : Math  Operator=log
  Exp1 : Math  Operator=log
  Multiply : Gain  Gain=1.87e-4
  Multiply1 : Gain  Gain=7.4e-5
  Multiply2 : Gain  Gain=3.12e-3
  Product : Product
  Product1 : Product
  Sum6 : Sum  Inputs=|-+-+
  n_act : Outport
  wires:
  T/1 -> Product1/2, Product/2, Multiply2/1
  Product1/1 -> Sum6/4
  Constant3/1 -> Sum6/1
  Con_O2/1 -> Exp1/1
  Exp1/1 -> Multiply1/1
  I/1 -> Exp/1
  Exp/1 -> Multiply/1
  Multiply1/1 -> Product1/1
  Multiply/1 -> Product/1
  Multiply2/1 -> Sum6/2
  Sum6/1 -> n_act/1
  Product/1 -> Sum6/3
